simulink model "stateSpaceControl5gdl"  (R2022b)
settings: Solver=VariableStepAuto  StartTime=0.0  StopTime=10.0  RelTol=1e-3
values from neighbouring files (symbols this model uses):
  cg_nom = 0.567    [linealizacion_5gdl.m]    (also in linealizacion_HEMS.m)
  Ka = [34.5916764023 4.46928641015 34.7816336405 4.65924364837 92.2484067139 -92.2484067139 74.2332308826 -74.2332308826 -4220.94514487 -4209.6309051 -4205.06787146 -4193.7536317 ... (120 elements, 8x15)]    [Ka.mat]    (also in linealizacion_5gdl_bien.m = place(Aa,Ba,[ -1.5 -1.5 -1.5 -1.5 -2 -2 -6 -6 -7 -7 -5 -5 -2; linealizacion_EMS.m = place(Aa,Ba,[ -1 -1 -2 -2 -3 -3 -6 -6 -7 -7 -5 -5 -4 -4 -5 -)
settings Model: Creator=USUARIO  LastModifiedBy=USUARIO

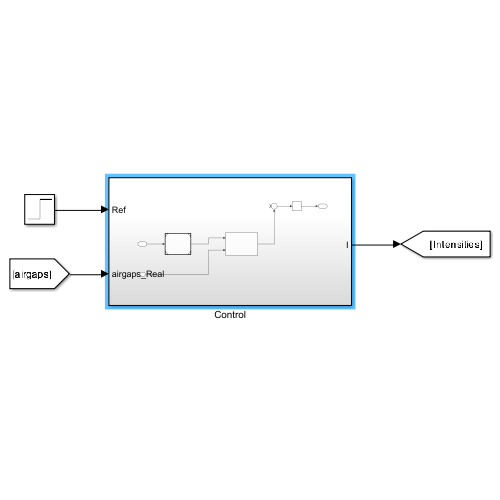
[thumbnail: Simulink's stored preview of the top-level diagram]
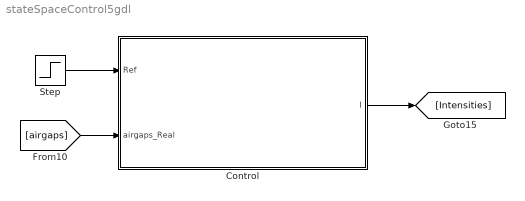
== system stateSpaceControl5gdl ==
  Control : Subsystem
  Step : Step  SampleTime=0
  wires:
  Step/1 -> Control/1(Ref)
  [airgaps] -> Control/2(airgaps_Real)
  Control/1(I) -> [Intensities]

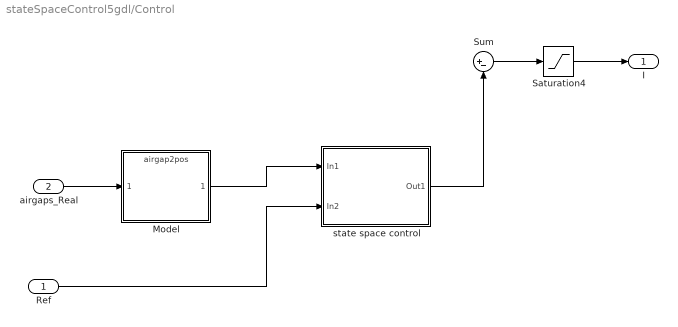
== system stateSpaceControl5gdl/Control ==
  Ref : Inport
  airgaps_Real : Inport  Port=2
  Model : ModelReference  ModelNameDialog=airgap2pos.slx  SimulationMode=Normal  ModelReferenceVersion=1.3
  Saturation4 : Saturate  UpperLimit=55  LowerLimit=-55
  Sum : Sum  Inputs=|+-
  state space control : Subsystem
  I : Outport
  wires:
  airgaps_Real/1 -> Model/1
  Sum/1 -> Saturation4/1
  Saturation4/1 -> I/1
  Model/1 -> state space control/1(In1)
  state space control/1(Out1) -> Sum/2
  Ref/1 -> state space control/2(In2)

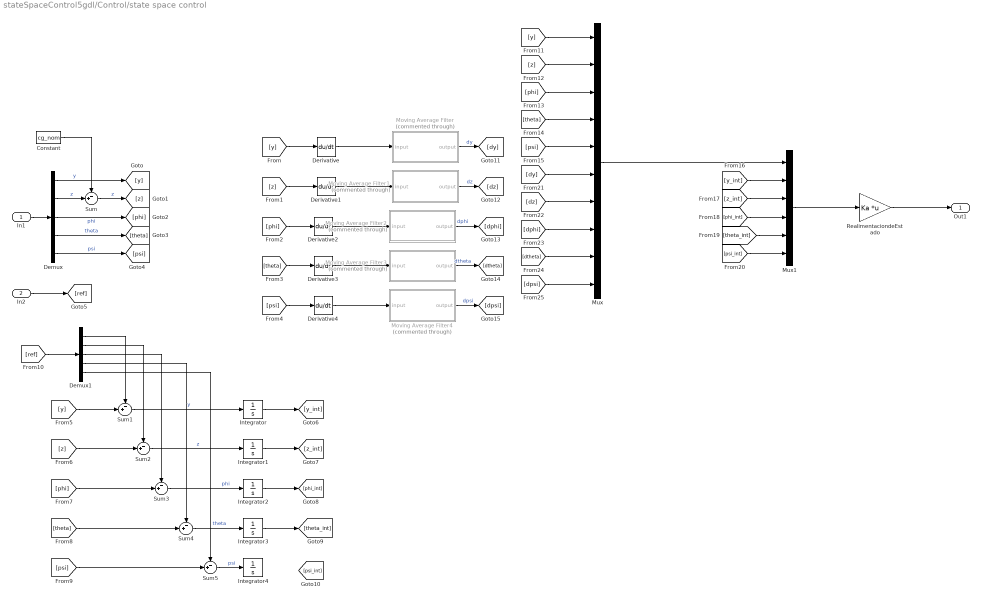
== system stateSpaceControl5gdl/Control/state space control ==
  In1 : Inport
  In2 : Inport  Port=2
  Constant : Constant  Value=cg_nom
  Demux : Demux  Outputs=5
  Demux1 : Demux  Outputs=5
  Derivative{,1..4} (5 alike) : Derivative
  Integrator{,1..4} (5 alike) : Integrator
  Moving Average Filter : Subsystem  Commented=through  mask{M=4, fs=-1}
      mask prompts: M "Orden del filtro (M)"; fs "Frecuencia de muestreo (fs)"
  Moving Average Filter1 : Subsystem  Commented=through  mask{M=4, fs=-1}
      mask prompts: M "Orden del filtro (M)"; fs "Frecuencia de muestreo (fs)"
  Moving Average Filter2 : Subsystem  Commented=through  mask{M=4, fs=-1}
      mask prompts: M "Orden del filtro (M)"; fs "Frecuencia de muestreo (fs)"
  Moving Average Filter3 : Subsystem  Commented=through  mask{M=4, fs=-1}
      mask prompts: M "Orden del filtro (M)"; fs "Frecuencia de muestreo (fs)"
  Moving Average Filter4 : Subsystem  Commented=through  mask{M=4, fs=-1}
      mask prompts: M "Orden del filtro (M)"; fs "Frecuencia de muestreo (fs)"
  Mux : Mux  Inputs=10
  Mux1 : Mux  Inputs=6
  RealimentaciondeEstado : Gain  Gain=Ka  Multiplication=Matrix(K*u)
  Sum{,1..5} (6 alike) : Sum  Inputs=-+|
  Out1 : Outport
  wires:
  In1/1 -> Demux/1
  RealimentaciondeEstado/1 -> Out1/1
  Derivative/1 -> Moving Average Filter/1(input)
  Derivative1/1 -> Moving Average Filter1/1(input)
  Derivative2/1 -> Moving Average Filter2/1(input)
  Derivative3/1 -> Moving Average Filter3/1(input)
  Derivative4/1 -> Moving Average Filter4/1(input)
  Mux/1 -> Mux1/1
  Demux/1 -> [y]  "y"
  Constant/1 -> Sum/1
  Sum/1 -> [z]  "z"
  Demux/2 -> Sum/2  "z"
  Demux/3 -> [phi]  "phi"
  Demux/4 -> [theta]  "theta"
  Demux/5 -> [psi]  "psi"
  [psi] -> Derivative4/1
  [theta] -> Derivative3/1
  [phi] -> Derivative2/1
  [z] -> Derivative1/1
  [y] -> Derivative/1
  In2/1 -> [ref]
  [ref] -> Demux1/1
  [y] -> Sum1/2
  [z] -> Sum2/2
  [phi] -> Sum3/2
  [theta] -> Sum4/2
  [psi] -> Sum5/2
  Demux1/1 -> Sum1/1
  Demux1/2 -> Sum2/1
  Demux1/3 -> Sum3/1
  Demux1/4 -> Sum4/1
  Demux1/5 -> Sum5/1
  Sum1/1 -> Integrator/1  "y"
  Sum5/1 -> Integrator4/1  "psi"
  Sum4/1 -> Integrator3/1  "theta"
  Sum3/1 -> Integrator2/1  "phi"
  Sum2/1 -> Integrator1/1  "z"
  [y] -> Mux/1
  [z] -> Mux/2
  [phi] -> Mux/3
  [theta] -> Mux/4
  [psi] -> Mux/5
  Integrator/1 -> [y_int]
  Integrator1/1 -> [z_int]
  Integrator2/1 -> [phi_int]
  Integrator3/1 -> [theta_int]
  Moving Average Filter/1(output) -> [dy]  "dy"
  Moving Average Filter1/1(output) -> [dz]  "dz"
  Moving Average Filter2/1(output) -> [dphi]  "dphi"
  Moving Average Filter4/1(output) -> [dpsi]  "dpsi"
  Moving Average Filter3/1(output) -> [dtheta]  "dtheta"
  [dpsi] -> Mux/10
  [dtheta] -> Mux/9
  [dphi] -> Mux/8
  [dz] -> Mux/7
  [dy] -> Mux/6
  [y_int] -> Mux1/2
  [psi_int] -> Mux1/6
  [theta_int] -> Mux1/5
  [phi_int] -> Mux1/4
  [z_int] -> Mux1/3
  Mux1/1 -> RealimentaciondeEstado/1

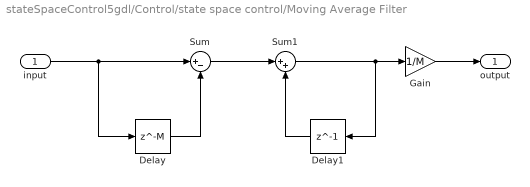
== system stateSpaceControl5gdl/Control/state space control/Moving Average Filter ==
  input : Inport
  Delay : Delay  DelayLength=M  SampleTime=fs
  Delay1 : Delay  DelayLength=1  SampleTime=fs
  Gain : Gain  Gain=1/M
  Sum : Sum  Inputs=|+-
  Sum1 : Sum  Inputs=|++
  output : Outport
  wires:
  input/1 -> Delay/1, Sum/1
  Delay/1 -> Sum/2
  Sum/1 -> Sum1/1
  Sum1/1 -> Delay1/1, Gain/1
  Delay1/1 -> Sum1/2
  Gain/1 -> output/1

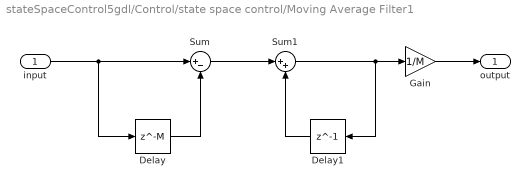
== system stateSpaceControl5gdl/Control/state space control/Moving Average Filter1 ==
  input : Inport
  Delay : Delay  DelayLength=M  SampleTime=fs
  Delay1 : Delay  DelayLength=1  SampleTime=fs
  Gain : Gain  Gain=1/M
  Sum : Sum  Inputs=|+-
  Sum1 : Sum  Inputs=|++
  output : Outport
  wires:
  input/1 -> Delay/1, Sum/1
  Delay/1 -> Sum/2
  Sum/1 -> Sum1/1
  Sum1/1 -> Delay1/1, Gain/1
  Delay1/1 -> Sum1/2
  Gain/1 -> output/1

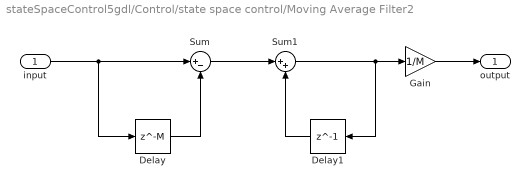
== system stateSpaceControl5gdl/Control/state space control/Moving Average Filter2 ==
  input : Inport
  Delay : Delay  DelayLength=M  SampleTime=fs
  Delay1 : Delay  DelayLength=1  SampleTime=fs
  Gain : Gain  Gain=1/M
  Sum : Sum  Inputs=|+-
  Sum1 : Sum  Inputs=|++
  output : Outport
  wires:
  input/1 -> Delay/1, Sum/1
  Delay/1 -> Sum/2
  Sum/1 -> Sum1/1
  Sum1/1 -> Delay1/1, Gain/1
  Delay1/1 -> Sum1/2
  Gain/1 -> output/1

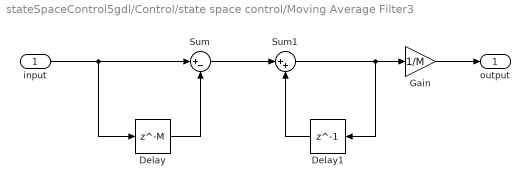
== system stateSpaceControl5gdl/Control/state space control/Moving Average Filter3 ==
  input : Inport
  Delay : Delay  DelayLength=M  SampleTime=fs
  Delay1 : Delay  DelayLength=1  SampleTime=fs
  Gain : Gain  Gain=1/M
  Sum : Sum  Inputs=|+-
  Sum1 : Sum  Inputs=|++
  output : Outport
  wires:
  input/1 -> Delay/1, Sum/1
  Delay/1 -> Sum/2
  Sum/1 -> Sum1/1
  Sum1/1 -> Delay1/1, Gain/1
  Delay1/1 -> Sum1/2
  Gain/1 -> output/1

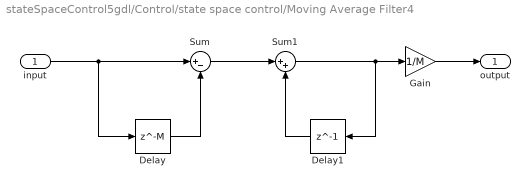
== system stateSpaceControl5gdl/Control/state space control/Moving Average Filter4 ==
  input : Inport
  Delay : Delay  DelayLength=M  SampleTime=fs
  Delay1 : Delay  DelayLength=1  SampleTime=fs
  Gain : Gain  Gain=1/M
  Sum : Sum  Inputs=|+-
  Sum1 : Sum  Inputs=|++
  output : Outport
  wires:
  input/1 -> Delay/1, Sum/1
  Delay/1 -> Sum/2
  Sum/1 -> Sum1/1
  Sum1/1 -> Delay1/1, Gain/1
  Delay1/1 -> Sum1/2
  Gain/1 -> output/1
